simulink model "exercise3_SIM"  (R2025b)
settings: Solver=VariableStepAuto  StartTime=0.0  StopTime=50  RelTol=1e-3
undefined symbols (not defined in the file or in its folder): par1, par2
libraries: cstblocks x1
settings Model: Creator=aless  LastModifiedBy=fred

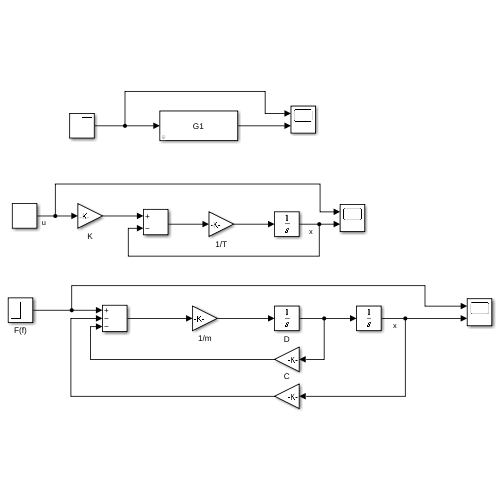
[thumbnail: Simulink's stored preview of the top-level diagram]
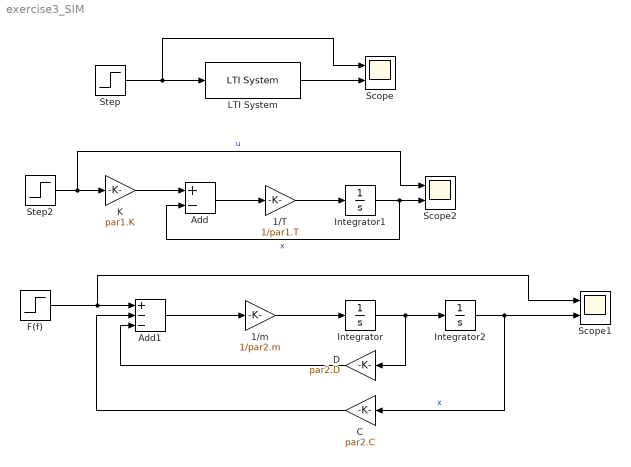
== system exercise3_SIM ==
  1/T : Gain  Gain=1/par1.T
  1/m : Gain  Gain=1/par2.m
  Add : Sum  Inputs=+-
  Add1 : Sum  Inputs=+--
  C : Gain  Gain=par2.C
  D : Gain  Tag=HHHH  Gain=par2.D
  F(f) : Step  SampleTime=0
  Integrator : Integrator
  Integrator1 : Integrator
  Integrator2 : Integrator
  K : Gain  Gain=par1.K
  LTI System : cstblocks/LTI System  sys=G1  IC=[]  PadeOrder=0
  Scope : Scope  NumInputPorts=2
      settings: ActiveDisplayYMinimum=-0.625  ActiveDisplayYMaximum=5.62497  DataLoggingVariableName=plotG1_Tf
  Scope1 : Scope  NumInputPorts=2
      settings: ActiveDisplayYMinimum=0.00019  ActiveDisplayYMaximum=0.01863  DataLoggingVariableName=plotE2
  Scope2 : Scope  NumInputPorts=2
      settings: ActiveDisplayYMinimum=-0.62499700930049706  ActiveDisplayYMaximum=5.6249730837044742  DataLoggingVariableName=plotG1_De
  Step : Step  SampleTime=0
  Step2 : Step  SampleTime=0
  wires:
  LTI System/1 -> Scope/2
  Step/1 -> Scope/1, LTI System/1
  Step2/1 -> Scope2/1, K/1  "u"
  K/1 -> Add/1
  Add/1 -> 1/T/1
  1/T/1 -> Integrator1/1
  Integrator1/1 -> Add/2, Scope2/2  "x"
  Integrator/1 -> D/1, Integrator2/1
  Integrator2/1 -> C/1, Scope1/2  "x"
  1/m/1 -> Integrator/1
  Add1/1 -> 1/m/1
  D/1 -> Add1/3
  C/1 -> Add1/2
  F(f)/1 -> Scope1/1, Add1/1
